simulink model "FOQL_PDE_SimpleExample"  (R2020a)
settings: Solver=VariableStepAuto  StartTime=0.0  StopTime=13  FixedStep=0.01  MaxStep=0.01  RelTol=1e-3
libraries: PDECharactLib x1
settings Model: Creator=kc5492  LastModifiedBy=User
settings SolverCC: ZeroCrossAlgorithm=Adaptive
settings DataIOCC: ReturnWorkspaceOutputs=off
settings DebuggingCC: PregeneratedLibrarySubsystemCodeDiagnostic=none  ArithmeticOperatorsInVariantConditions=warning
settings SFSimCC: SimUseLocalCustomCode=off  CustomCodeUndefinedFunction=UseInterfaceOnly
settings RTWCC: RTWUseLocalCustomCode=off

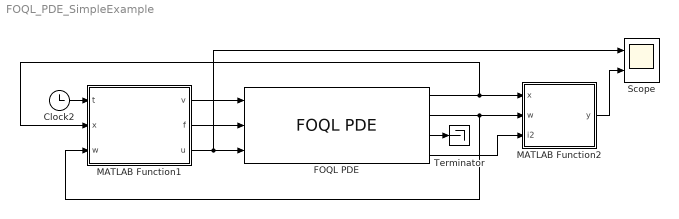
== system FOQL_PDE_SimpleExample ==
  Clock2 : Clock
  FOQL PDE : PDECharactLib/FOQL PDE  ell=1  Nmax=100  x0=0:0.1:1  w0=1 - (0:0.1:1).^2  initX=0  initW=0  dx=0.1  dw=0.1  dt=0.1  crossing_tol=1e-11  overflow_err=off
  MATLAB Function1 : MATLAB Function  TreatAsAtomicUnit=on
  MATLAB Function2 : MATLAB Function  TreatAsAtomicUnit=on
  Scope : Scope  NumInputPorts=2
  Terminator : Terminator
  wires:
  Clock2/1 -> MATLAB Function1/1(t)
  FOQL PDE/1 -> MATLAB Function1/2(x), MATLAB Function2/1(x)
  FOQL PDE/2 -> MATLAB Function1/3(w), MATLAB Function2/2(w)
  FOQL PDE/4 -> MATLAB Function2/3(i2)
  FOQL PDE/3 -> Terminator/1
  MATLAB Function1/1(v) -> FOQL PDE/1
  MATLAB Function1/2(f) -> FOQL PDE/2
  MATLAB Function1/3(u) -> Scope/1, FOQL PDE/3
  MATLAB Function2/1(y) -> Scope/2

== matlab function FOQL_PDE_SimpleExample/MATLAB Function1 ==
  data: t input; v output; x input; w input; f output; u output
function [v, f, u] = equationTerms(t, x, w)

v = x + 1.1 + sin(t);
f = -w;
u = (t <= 16) * (1 + cos(pi/2*t))/2;

== matlab function FOQL_PDE_SimpleExample/MATLAB Function2 ==
  data: x input; y output; w input; i2 input
function y = output(x, w, i2)

if i2 == 1
    i2prev = length(x);
else
    i2prev = i2 - 1;
end

% Domain length = 1
y = w(i2prev) + (w(i2) - w(i2prev))/(x(i2) - x(i2prev))*(1 - x(i2prev));
